simulink model "part3"  (R2018a)
settings: Solver=VariableStepAuto  StartTime=0.0  StopTime=20  RelTol=1e-3
undefined symbols (not defined in the file or in its folder): cd, gc, m
settings Model: Creator=jschm  LastModifiedBy=jschm

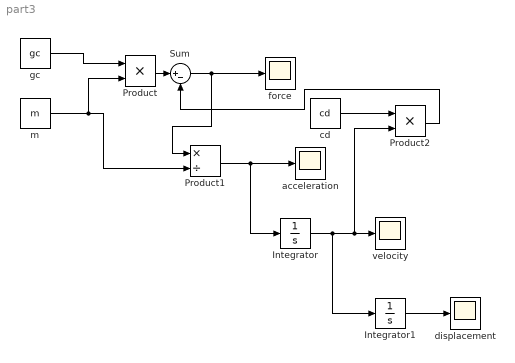
== system part3 ==
  Integrator : Integrator  InitialCondition=200
  Integrator1 : Integrator  InitialCondition=10
  Product : Product
  Product1 : Product  Inputs=*/
  Product2 : Product
  Sum : Sum  Inputs=|+-
  acceleration : Scope
  cd : Constant  Value=cd
  displacement : Scope
  force : Scope
  "gc " : Constant  Value=gc
  m : Constant  Value=m
  velocity : Scope
  wires:
  "gc "/1 -> Product/1
  Product/1 -> Sum/1
  m/1 -> Product/2, Product1/2
  Product1/1 -> Integrator/1, acceleration/1
  Integrator/1 -> Integrator1/1, Product2/2, velocity/1
  Integrator1/1 -> displacement/1
  Sum/1 -> Product1/1, force/1
  cd/1 -> Product2/1
  Product2/1 -> Sum/2
